simulink model "EncodersVelocidad"  (R2023b)
settings: Solver=VariableStepAuto  StartTime=0.0  StopTime=10.0  RelTol=1e-3
libraries: arduinosensorlib x2
settings Model: Creator=pcele  LastModifiedBy=pcele

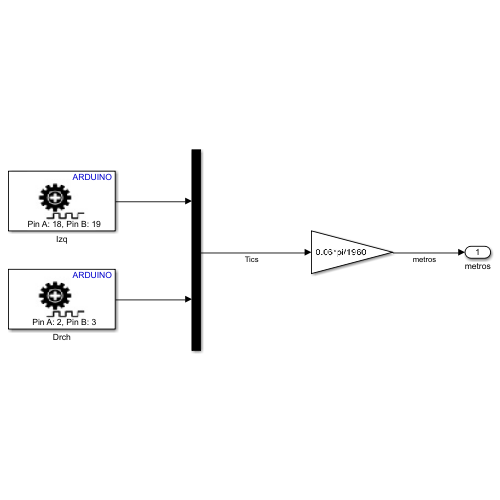
[thumbnail: Simulink's stored preview of the top-level diagram]
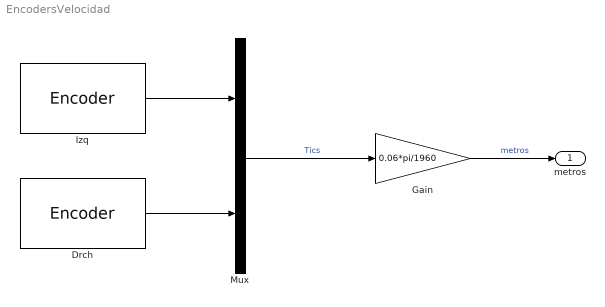
== system EncodersVelocidad ==
  Drch : arduinosensorlib/Encoder  InputA=2  InputB=3  Mode=No reset  SampleTime=-1
  Gain : Gain  Gain=0.06*pi/1960  ParamDataTypeStr=double
  Izq : arduinosensorlib/Encoder  InputA=18  InputB=19  Mode=No reset  SampleTime=-1
  Mux : Mux  Inputs=2
  metros : Outport
  wires:
  Mux/1 -> Gain/1  "Tics"
  Gain/1 -> metros/1  "metros"
  Drch/1 -> Mux/2
  Izq/1 -> Mux/1
